simulink model "codesAnalyseHadamard"  (R2012b)
settings: Solver=ode45  StartTime=0.0  StopTime=10.0  RelTol=1e-3
undefined symbols (not defined in the file or in its folder): get
libraries: dspstat3 x2, commseqgen2 x2, dspsnks4 x2
settings Model: Creator=mcaceres  LastModifiedBy=mcaceres

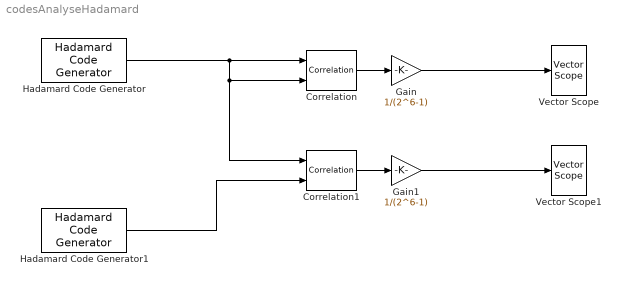
== system codesAnalyseHadamard ==
  Correlation : dspstat3/Correlation  domain=Time  outputDataTypeStr=Inherit: Same as accumulator  outputLastDataTypeStr=Inherit: Same as accumulator  outputMin=[]  outputMax=[]  roundingMode=Floor  overflowMode=off
  Correlation1 : dspstat3/Correlation  domain=Time  outputDataTypeStr=Inherit: Same as accumulator  outputLastDataTypeStr=Inherit: Same as accumulator  outputMin=[]  outputMax=[]  roundingMode=Floor  overflowMode=off
  Gain : Gain  Gain=1/(2^6-1)
  Gain1 : Gain  Gain=1/(2^6-1)
  Hadamard Code Generator : commseqgen2/Hadamard Code Generator  length=128  index=60  ts=10^-6/128  frameBased=on  sampPerFrame=128  outDataType=double
  Hadamard Code Generator1 : commseqgen2/Hadamard Code Generator  length=128  index=50  ts=10^-6/128  frameBased=on  sampPerFrame=128  outDataType=double
  Vector Scope : dspsnks4/Vector Scope  ScopeProperties=on  Domain=Time  HorizSpan=1  DisplayProperties=off  AxisGrid=on  Memory=off  FrameNumber=on  AxisLegend=off  AxisZoom=off  OpenScopeAtSimStart=on  OpenScopeImmediately=off  FigPos=get(0,'defaultfigureposition')  AxisProperties=off  XUnits=Hertz  XRange=[0...Fs/2]  InheritXIncr=on  XIncr=1  XLabel=Time  XLimit=Auto  XMin=0  XMax=1  XStart=0  YUnits=dB  YLabel=Amplitude  LineProperties=off  XAxisParamsVer=6.9
      settings: YMin=-10  YMax=10
  Vector Scope1 : dspsnks4/Vector Scope  ScopeProperties=on  Domain=Time  HorizSpan=1  DisplayProperties=off  AxisGrid=on  Memory=off  FrameNumber=on  AxisLegend=off  AxisZoom=off  OpenScopeAtSimStart=on  OpenScopeImmediately=off  FigPos=get(0,'defaultfigureposition')  AxisProperties=off  XUnits=Hertz  XRange=[0...Fs/2]  InheritXIncr=on  XIncr=1  XLabel=Time  XLimit=Auto  XMin=0  XMax=1  XStart=0  YUnits=dB  YLabel=Amplitude  LineProperties=off  XAxisParamsVer=6.9
      settings: YMin=-10  YMax=10
  wires:
  Correlation/1 -> Gain/1
  Correlation1/1 -> Gain1/1
  Gain/1 -> Vector Scope/1
  Gain1/1 -> Vector Scope1/1
  Hadamard Code Generator1/1 -> Correlation1/2
  Hadamard Code Generator/1 -> Correlation1/1, Correlation/2, Correlation/1
